simulink model "chua_c_sim_2014"  (R2014a)
settings: Solver=ode23t  SolverMode=SingleTasking  StartTime=0.0  StopTime=Tfin  RelTol=1e-3
values from neighbouring files (symbols this model uses):
  ie = 1    [main_chua.m]
  K = place(A{ie},g,[-1,-2,-3])    [main_chua.m]
  x0 = randn(3,1)*0.2    [main_chua.m]
undefined symbols (not defined in the file or in its folder): fg_chua, xeq
settings Model: CovMetricSettings=dwe  CovHtmlReporting=off  covSaveCumulativeToWorkspaceVar=off  CovSaveSingleToWorkspaceVar=off  CovExternalEMLEnable=on  CovSFcnEnable=on  Creator=carlonovara  LastModifiedBy=carlonovara
settings DataIOCC: LimitDataPoints=off  SaveFormat=StructureWithTime
settings DebuggingCC: MergeDetectMultiDrivingBlocksExec=error  SolverPrmCheckMsg=none  FrameProcessingCompatibilityMsg=error  SFUnexpectedBacktrackingDiag=error  SFNoUnconditionalDefaultTransitionDiag=error
settings HardwareCC: ProdBitPerPointer=64  ProdLargestAtomicFloat=Float  ProdIntDivRoundTo=Zero  ProdEndianess=LittleEndian  ProdHWDeviceType=Specified
settings ModelReferenceCC: PropagateSignalLabelsOutOfModel=on
settings GRTTargetCC: TargetLangStandard=C99 (ISO)  GeneratePreprocessorConditionals=Use local settings

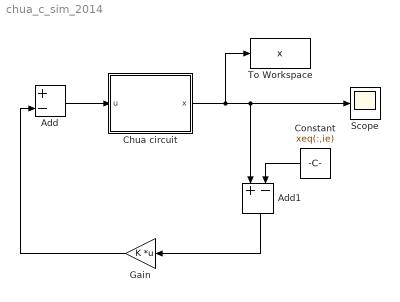
== system chua_c_sim_2014 ==
  Add : Sum  Inputs=+-
  Add1 : Sum  Inputs=+-
  Chua circuit : Subsystem
  Constant : Constant  Value=xeq(:,ie)
  Gain : Gain  Gain=K  Multiplication=Matrix(K*u)
  Scope : Scope
      settings: TimeRange=auto  MaxDataPoints=5000  SaveToWorkspace=off  SaveName=ScopeData  YMin=-0.37601  YMax=0.36722  SampleTime=-1
  To Workspace : ToWorkspace  VariableName=x  SampleTime=-1
  wires:
  Chua circuit/1(x) -> Scope/1, Add1/1, To Workspace/1
  Add/1 -> Chua circuit/1(u)
  Gain/1 -> Add/2
  Add1/1 -> Gain/1
  Constant/1 -> Add1/2

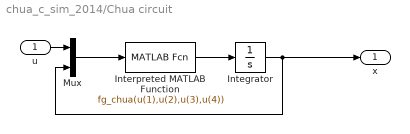
== system chua_c_sim_2014/Chua circuit ==
  u : Inport
  Integrator : Integrator  InitialCondition=x0
  Interpreted MATLAB Function : MATLABFcn  MATLABFcn=fg_chua(u(1),u(2),u(3),u(4))  OutputDimensions=3
  Mux : Mux  Inputs=2
  x : Outport
  wires:
  u/1 -> Mux/1
  Interpreted MATLAB Function/1 -> Integrator/1
  Integrator/1 -> Mux/2, x/1
  Mux/1 -> Interpreted MATLAB Function/1
